simulink library "lib_Sim_CRM_16b"  (Simulink 8.8)
settings: Solver=VariableStepAuto  StartTime=0.0  StopTime=10.0  RelTol=1e-3
undefined symbols (not defined in the file): CRM
libraries: simulink x1
settings Model: Creator=cava_da  LastModifiedBy=cava_da

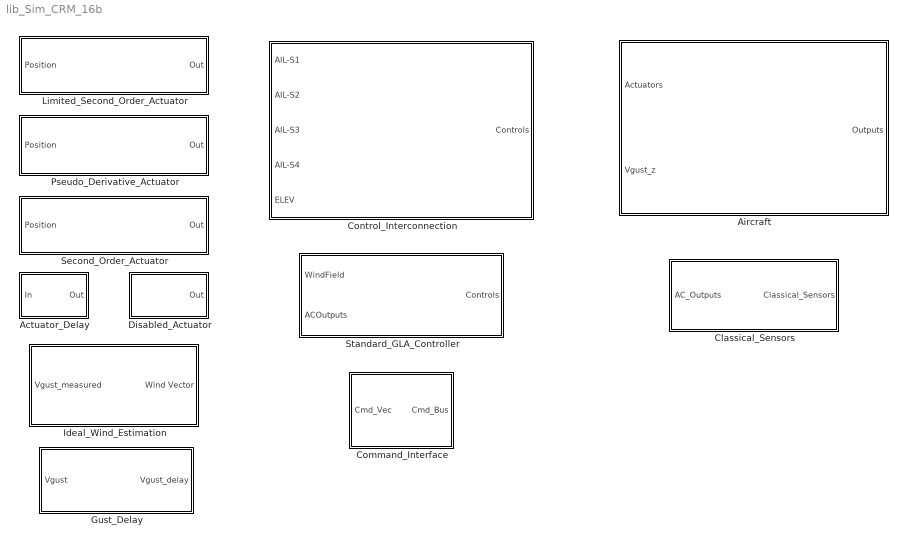
== system lib_Sim_CRM_16b ==
  Actuator_Delay : Subsystem  mask(Actuator Delay){Act_Delay=CRM.Actuators.Global_Delay}
      mask prompts: Act_Delay "Insert actuator delay [s]"
      mask help: Applies a transport delay to actuator commands.
      mask Display:
      | port_label('input', 1, '')
      | port_label('output',1, '')
  Aircraft : Subsystem  mask(Aircraft model){modelName=CRM.Aircraft}
      mask prompts: modelName "Insert name of model parameter struct (e.g. CRM.Aircraft):"
      mask help:
      | Contains the state-space model of the aircraft, separates the outputs and
      | measurements, as specified.
      mask Display:
      | port_label('input', 2, 'Gust')
      | port_label('input', 1, 'Actuators')
      | port_label('output', 1, 'Outputs')
  Classical_Sensors : Subsystem
  Command_Interface : Subsystem
  Control_Interconnection : Subsystem  mask(Control interconnection block){}
      mask help:
      | Accepts actuator states in the form of a bus containing position, rate,
      | and acceleration (delta, deltadot, delta2dot, respectively) for each
      | actuator, and rearranges them in the order required by the model.
      mask Display:
      | image(imread('plane_actuators_color.png'))
      | port_label('output', 1, 'Actuators')
      | port_label('input', 1, 'S1')
      | port_label('input', 2, 'S2')
      | port_label('input', 3, 'S3')
      | port_label('input', 4, 'S4')
      | port_label('input', 5, 'ELEV')
  Disabled_Actuator : Subsystem  mask(Disabled Actuator){}
      mask help:
      | Generates a bus containing actuator position,
      | rate, and acceleration equal to zero.
      mask Display:
      | port_label('output',1, 'Pos/Rate/Acc')
      | text(0.5,0.1, 'DA', 'horizontalAlignment', 'center')
  Gust_Delay : Subsystem  mask(Gust delay block){weName=CRM.WindEst}
      mask prompts: weName "Insert the wind estimation struct (e.g. CRM.WindEst):"
      mask help:
      | Delays the gust input so that it 'arrives' at the aircraft nose with the
      | appropriate delay w.r.t. the LIDAR/Wind Estimator prediction.
      mask Display:
      | port_label('input', 1, 'Measured gust')
      | port_label('output', 1, 'Delayed gust')
  Ideal_Wind_Estimation : Subsystem  mask(Wind Estimation Block){weName=CRM.WindEst}
      mask prompts: weName "Insert the wind estimation struct (e.g. CRM.WindEst):"
      mask help:
      | Accepts wind speed (measured by LIDAR) and generates the delayed vector of
      | estimated wind speeds.
      | The wind vector is ordered from oldest (i.e. at aircraft position) to newest
      | (i.e. currently measured by LIDAR).
      mask Display:
      | port_label('input', 1, 'Measured Wind')
      | port_label('output', 1, 'Wind Vector')
  Limited_Second_Order_Actuator : Subsystem  mask(Second-Order Actuator){actuatorName=CRM.Actuators.OuterAileron}
      mask prompts: actuatorName "Insert actuator struct (e.g. CRM.Actuators.OuterAileron):"
      mask help:
      | Accepts a commanded actuator position, and
      | generates a bus containing actuator position,
      | rate, and acceleration.
      |
      | This block uses a 2nd-order linear system to
      | approximate an actuation loop.
      mask Display:
      | port_label('input', 1, 'Commanded Pos')
      | port_label('output',1, 'Pos/Rate/Acc')
      | text(0.5,0.1, 'SO-LIM', 'horizontalAlignment', 'center')
  Pseudo_Derivative_Actuator : Subsystem  mask(Pseudo-derivative Actuator){actuatorName=CRM.Actuators.OuterAileron}
      mask prompts: actuatorName "Insert actuator struct (e.g. CRM.Actuators.Aileron):"
      mask help:
      | Accepts a commanded actuator position, and
      | generates a bus containing actuator position,
      | rate, and acceleration.
      |
      | This block uses 2 pseudo-derivatives to approximate this.
      mask Display:
      | port_label('input', 1, 'Commanded Pos')
      | port_label('output',1, 'Pos/Rate/Acc')
      | text(0.5,0.1, 'PD', 'horizontalAlignment', 'center')
  Second_Order_Actuator : Subsystem  mask(Second-Order Actuator){actuatorName=CRM.Actuators.OuterAileron}
      mask prompts: actuatorName "Insert actuator struct (e.g. CRM.Actuators.OuterAileron):"
      mask help:
      | Accepts a commanded actuator position, and
      | generates a bus containing actuator position,
      | rate, and acceleration.
      |
      | This block uses a 2nd-order linear system to
      | approximate an actuation loop.
      mask Display:
      | port_label('input', 1, 'Commanded Pos')
      | port_label('output',1, 'Pos/Rate/Acc')
      | text(0.5,0.1, 'SO', 'horizontalAlignment', 'center')
  Standard_GLA_Controller : Subsystem  mask(Simple Gust Load Alleviation Controller Block){glaName=CRM.GLA}
      mask prompts: glaName "Insert the GLA structure (e.g. CRM.GLA):"
      mask help:
      | Calculates control inputs based on measured variables, such as the lidar wind field.
      | This block assumes that the controller is contained in a single discrete state-space system.
      | The output contains 3 signals, in the following order:
      |    Inner Aileron, Outer Aileron, Elevator.
      | If the controller does not use one or more of them, it is automatically set to 0.
      mask Display:
      | port_label('input', 2, 'A/C Outputs')
      | port_label('input', 1, 'Wind Field')
      | port_label('output', 1, 'Controls')

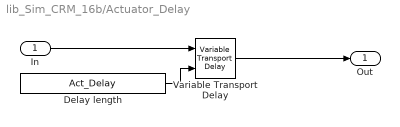
== system lib_Sim_CRM_16b/Actuator_Delay ==
  In : Inport
  Delay length : Constant  Value=Act_Delay
  Variable Transport Delay : VariableTransportDelay  MaximumDelay=Act_Delay  ZeroDelay=on
  Out : Outport
  wires:
  Variable Transport Delay/1 -> Out/1
  In/1 -> Variable Transport Delay/1
  Delay length/1 -> Variable Transport Delay/2

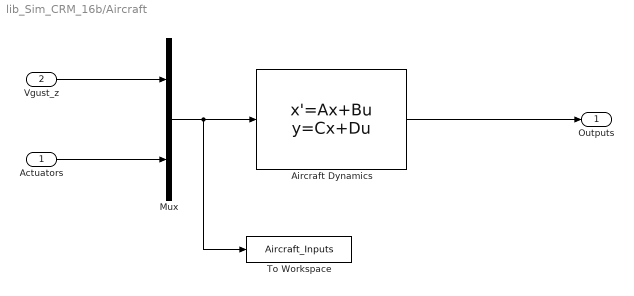
== system lib_Sim_CRM_16b/Aircraft ==
  Actuators : Inport
  Vgust_z : Inport  Port=2
  Aircraft Dynamics : StateSpace  A=modelName.linear_sys.A  B=modelName.linear_sys.B  C=[modelName.C_sensors; modelName.C_outputs]  D=[modelName.D_sensors; modelName.D_outputs]  X0=0
  Mux : Mux  Inputs=2
  To Workspace : ToWorkspace  VariableName=Aircraft_Inputs  SaveFormat=Structure With Time  SampleTime=-1
      settings: Decimation=SimConfig.Logging.DecimationFactor
  Outputs : Outport
  wires:
  Mux/1 -> To Workspace/1, Aircraft Dynamics/1
  Aircraft Dynamics/1 -> Outputs/1
  Vgust_z/1 -> Mux/1
  Actuators/1 -> Mux/2

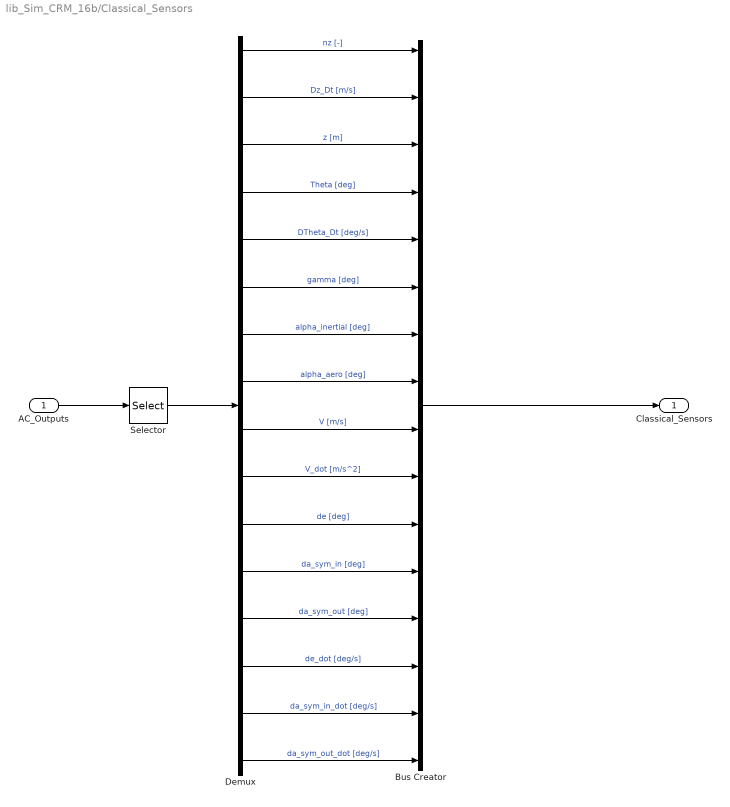
== system lib_Sim_CRM_16b/Classical_Sensors ==
  AC_Outputs : Inport
  Bus Creator : BusCreator  Inputs=16
  Demux : Demux  Outputs=16
  Selector : Selector  IndexOptions=Index vector (dialog)  Indices=1:CRM.Sensors.Classical.Num_Signals  OutputSizes=1
  Classical_Sensors : Outport
  wires:
  AC_Outputs/1 -> Selector/1
  Selector/1 -> Demux/1
  Demux/1 -> Bus Creator/1  "nz [-]"
  Demux/6 -> Bus Creator/6  "gamma [deg]"
  Demux/5 -> Bus Creator/5  "DTheta_Dt [deg/s]"
  Demux/7 -> Bus Creator/7  "alpha_inertial [deg]"
  Demux/4 -> Bus Creator/4  "Theta [deg]"
  Demux/8 -> Bus Creator/8  "alpha_aero [deg]"
  Demux/3 -> Bus Creator/3  "z [m]"
  Demux/9 -> Bus Creator/9  "V [m/s]"
  Demux/2 -> Bus Creator/2  "Dz_Dt [m/s]"
  Demux/10 -> Bus Creator/10  "V_dot [m/s^2]"
  Demux/11 -> Bus Creator/11  "de [deg]"
  Demux/12 -> Bus Creator/12  "da_sym_in [deg]"
  Demux/13 -> Bus Creator/13  "da_sym_out [deg]"
  Demux/14 -> Bus Creator/14  "de_dot [deg/s]"
  Demux/15 -> Bus Creator/15  "da_sym_in_dot [deg/s]"
  Demux/16 -> Bus Creator/16  "da_sym_out_dot [deg/s]"
  Bus Creator/1 -> Classical_Sensors/1

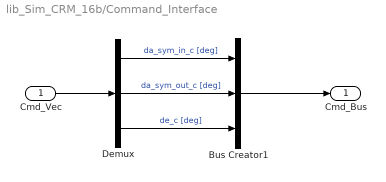
== system lib_Sim_CRM_16b/Command_Interface ==
  Cmd_Vec : Inport
  Bus Creator1 : BusCreator  Inputs=3
  Demux : Demux  Outputs=3
  Cmd_Bus : Outport
  wires:
  Demux/2 -> Bus Creator1/2  "da_sym_out_c [deg]"
  Demux/1 -> Bus Creator1/1  "da_sym_in_c [deg]"
  Demux/3 -> Bus Creator1/3  "de_c [deg]"
  Cmd_Vec/1 -> Demux/1
  Bus Creator1/1 -> Cmd_Bus/1

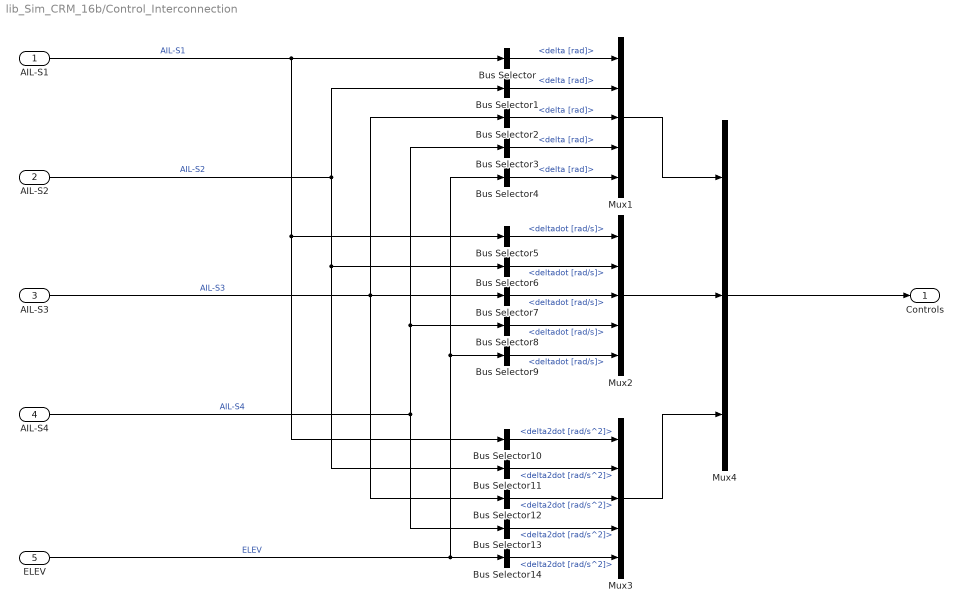
== system lib_Sim_CRM_16b/Control_Interconnection ==
  AIL-S1 : Inport
  AIL-S2 : Inport  Port=2
  AIL-S3 : Inport  Port=3
  AIL-S4 : Inport  Port=4
  ELEV : Inport  Port=5
  Bus Selector{,1..4} (5 alike) : BusSelector  OutputSignals=delta [rad]
  Bus Selector{10..14} (5 alike) : BusSelector  OutputSignals=delta2dot [rad/s^2]
  Bus Selector{5..9} (5 alike) : BusSelector  OutputSignals=deltadot [rad/s]
  Mux1 : Mux  Inputs=5
  Mux2 : Mux  Inputs=5
  Mux3 : Mux  Inputs=5
  Mux4 : Mux  Inputs=3
  Controls : Outport
  wires:
  Mux2/1 -> Mux4/2
  Mux1/1 -> Mux4/1
  Mux3/1 -> Mux4/3
  Bus Selector14/1 -> Mux3/5  "<delta2dot [rad/s^2]>"
  Bus Selector13/1 -> Mux3/4  "<delta2dot [rad/s^2]>"
  Bus Selector12/1 -> Mux3/3  "<delta2dot [rad/s^2]>"
  Bus Selector11/1 -> Mux3/2  "<delta2dot [rad/s^2]>"
  Bus Selector10/1 -> Mux3/1  "<delta2dot [rad/s^2]>"
  Bus Selector9/1 -> Mux2/5  "<deltadot [rad/s]>"
  Bus Selector8/1 -> Mux2/4  "<deltadot [rad/s]>"
  Bus Selector7/1 -> Mux2/3  "<deltadot [rad/s]>"
  Bus Selector6/1 -> Mux2/2  "<deltadot [rad/s]>"
  Bus Selector5/1 -> Mux2/1  "<deltadot [rad/s]>"
  Bus Selector4/1 -> Mux1/5  "<delta [rad]>"
  Bus Selector3/1 -> Mux1/4  "<delta [rad]>"
  Bus Selector2/1 -> Mux1/3  "<delta [rad]>"
  Bus Selector1/1 -> Mux1/2  "<delta [rad]>"
  Bus Selector/1 -> Mux1/1  "<delta [rad]>"
  AIL-S1/1 -> Bus Selector/1, Bus Selector5/1, Bus Selector10/1  "AIL-S1"
  AIL-S2/1 -> Bus Selector1/1, Bus Selector6/1, Bus Selector11/1  "AIL-S2"
  AIL-S3/1 -> Bus Selector2/1, Bus Selector7/1, Bus Selector12/1  "AIL-S3"
  Mux4/1 -> Controls/1
  AIL-S4/1 -> Bus Selector3/1, Bus Selector8/1, Bus Selector13/1  "AIL-S4"
  ELEV/1 -> Bus Selector4/1, Bus Selector9/1, Bus Selector14/1  "ELEV"

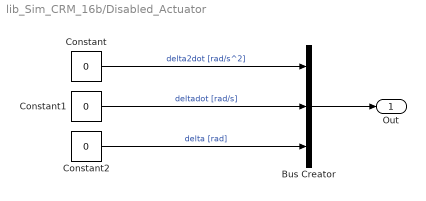
== system lib_Sim_CRM_16b/Disabled_Actuator ==
  Bus Creator : BusCreator  Inputs=3
  Constant : Constant  Value=0
  Constant1 : Constant  Value=0
  Constant2 : Constant  Value=0
  Out : Outport
  wires:
  Constant2/1 -> Bus Creator/3  "delta [rad]"
  Constant1/1 -> Bus Creator/2  "deltadot [rad/s]"
  Constant/1 -> Bus Creator/1  "delta2dot [rad/s^2]"
  Bus Creator/1 -> Out/1

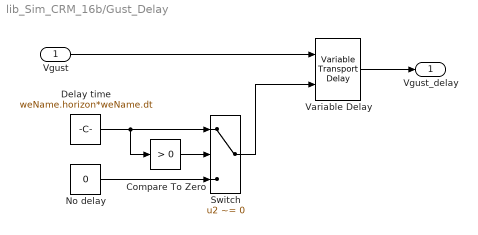
== system lib_Sim_CRM_16b/Gust_Delay ==
  Vgust : Inport
  Compare To Zero : simulink/Logic and Bit Operations/Compare To Zero  relop=>  OutDataTypeStr=uint8  ZeroCross=off
  Delay time : Constant  Value=weName.horizon*weName.dt
  No delay : Constant  Value=0
  Switch : Switch  Criteria=u2 ~= 0
  Variable Delay : VariableTransportDelay  MaximumDelay=10  MaximumPoints=1024*15  ZeroDelay=on  TransDelayFeedthrough=on
  Vgust_delay : Outport
  wires:
  Delay time/1 -> Switch/1, Compare To Zero/1
  Vgust/1 -> Variable Delay/1
  Variable Delay/1 -> Vgust_delay/1
  No delay/1 -> Switch/3
  Compare To Zero/1 -> Switch/2
  Switch/1 -> Variable Delay/2

== system lib_Sim_CRM_16b/Ideal_Wind_Estimation ==
  Vgust_measured : Inport
  Wind Estimator : DiscreteStateSpace  A=weName.A  B=weName.B  C=weName.C  D=weName.D  SampleTime=weName.dt
  Zero-Order Hold : ZeroOrderHold  SampleTime=weName.dt
  Wind Vector : Outport
  wires:
  Zero-Order Hold/1 -> Wind Estimator/1
  Wind Estimator/1 -> Wind Vector/1
  Vgust_measured/1 -> Zero-Order Hold/1

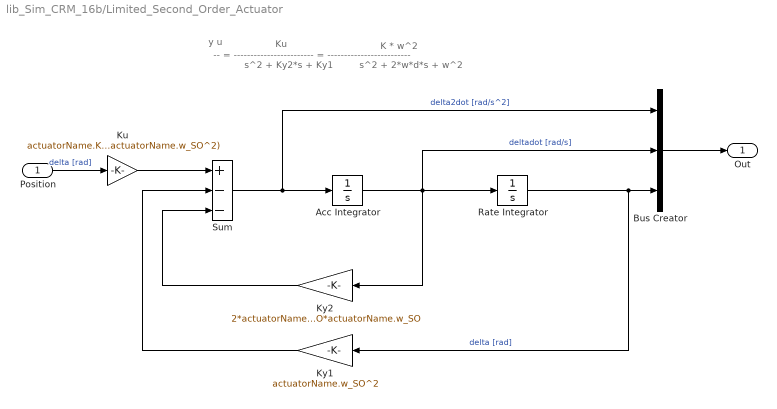
== system lib_Sim_CRM_16b/Limited_Second_Order_Actuator ==
  note: s^2 + 2*w*d*s + w^2
  note: K * w^2
  note: s^2 + Ky2*s + Ky1
  note: Ku
  note: -- = ------------------------ = -------------------------
  note: y
      |
      | u
  Position : Inport
  Acc Integrator : Integrator  LimitOutput=on  UpperSaturationLimit=actuatorName.rateLim  LowerSaturationLimit=-actuatorName.rateLim
  Bus Creator : BusCreator  Inputs=3
  Ku : Gain  Gain=actuatorName.K_st * (actuatorName.w_SO^2)
  Ky1 : Gain  Gain=actuatorName.w_SO^2
  Ky2 : Gain  Gain=2*actuatorName.d_SO*actuatorName.w_SO
  Rate Integrator : Integrator  LimitOutput=on  UpperSaturationLimit=actuatorName.posLim  LowerSaturationLimit=-actuatorName.posLim
  Sum : Sum  Inputs=+--
  Out : Outport
  wires:
  Ku/1 -> Sum/1
  Ky1/1 -> Sum/2
  Ky2/1 -> Sum/3
  Rate Integrator/1 -> Bus Creator/3, Ky1/1  "delta [rad]"
  Acc Integrator/1 -> Rate Integrator/1, Bus Creator/2, Ky2/1  "deltadot [rad/s]"
  Sum/1 -> Bus Creator/1, Acc Integrator/1  "delta2dot [rad/s^2]"
  Position/1 -> Ku/1  "delta [rad]"
  Bus Creator/1 -> Out/1

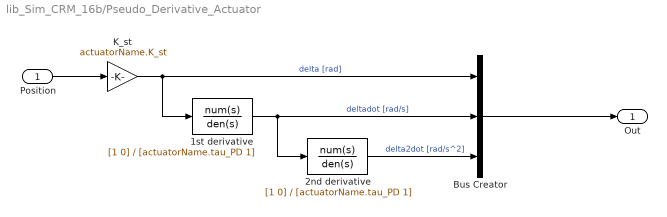
== system lib_Sim_CRM_16b/Pseudo_Derivative_Actuator ==
  Position : Inport
  1st derivative : TransferFcn  Numerator=[1 0]  Denominator=[actuatorName.tau_PD 1]
  2nd derivative : TransferFcn  Numerator=[1 0]  Denominator=[actuatorName.tau_PD 1]
  Bus Creator : BusCreator  Inputs=3
  K_st : Gain  Gain=actuatorName.K_st
  Out : Outport
  wires:
  1st derivative/1 -> 2nd derivative/1, Bus Creator/2  "deltadot [rad/s]"
  Position/1 -> K_st/1
  2nd derivative/1 -> Bus Creator/3  "delta2dot [rad/s^2]"
  Bus Creator/1 -> Out/1
  K_st/1 -> 1st derivative/1, Bus Creator/1  "delta [rad]"

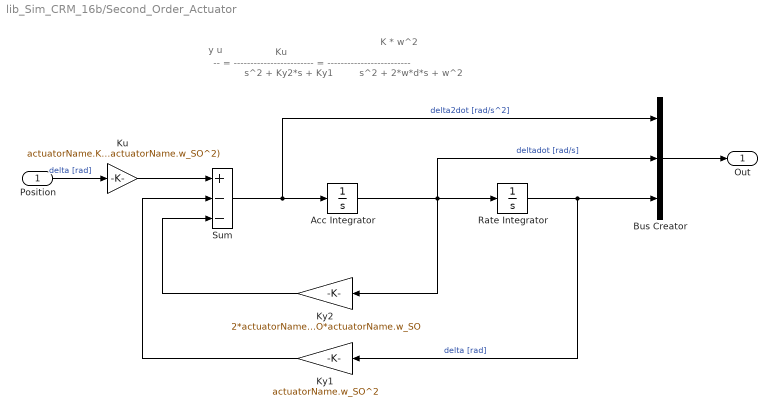
== system lib_Sim_CRM_16b/Second_Order_Actuator ==
  note: y
      |
      | u
  note: -- = ------------------------ = -------------------------
  note: Ku
  note: s^2 + Ky2*s + Ky1
  note: K * w^2
  note: s^2 + 2*w*d*s + w^2
  Position : Inport
  Acc Integrator : Integrator
  Bus Creator : BusCreator  Inputs=3
  Ku : Gain  Gain=actuatorName.K_st * (actuatorName.w_SO^2)
  Ky1 : Gain  Gain=actuatorName.w_SO^2
  Ky2 : Gain  Gain=2*actuatorName.d_SO*actuatorName.w_SO
  Rate Integrator : Integrator
  Sum : Sum  Inputs=+--
  Out : Outport
  wires:
  Bus Creator/1 -> Out/1
  Position/1 -> Ku/1  "delta [rad]"
  Sum/1 -> Acc Integrator/1, Bus Creator/1  "delta2dot [rad/s^2]"
  Acc Integrator/1 -> Rate Integrator/1, Ky2/1, Bus Creator/2  "deltadot [rad/s]"
  Rate Integrator/1 -> Ky1/1, Bus Creator/3  "delta [rad]"
  Ky2/1 -> Sum/3
  Ky1/1 -> Sum/2
  Ku/1 -> Sum/1

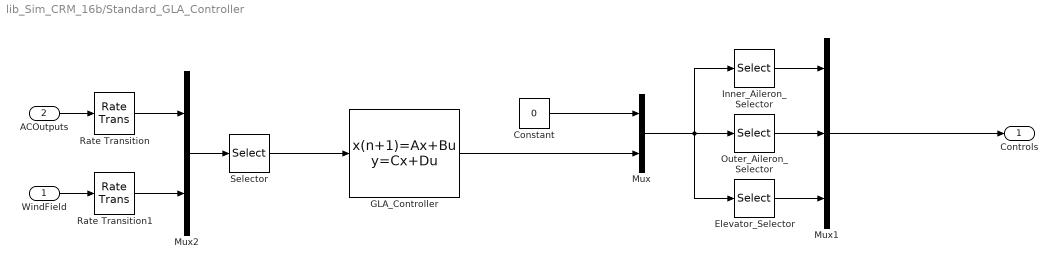
== system lib_Sim_CRM_16b/Standard_GLA_Controller ==
  WindField : Inport
  ACOutputs : Inport  Port=2
  Constant : Constant  Value=0
  Elevator_Selector : Selector  IndexMode=Zero-based  IndexOptions=Index vector (dialog)  Indices=[glaName.de_idx]  OutputSizes=1
  GLA_Controller : DiscreteStateSpace  A=glaName.A  B=glaName.B  C=glaName.C  D=glaName.D  SampleTime=glaName.dt
  Inner_Aileron_Selector : Selector  IndexMode=Zero-based  IndexOptions=Index vector (dialog)  Indices=[glaName.dain_idx]  OutputSizes=1
  Mux : Mux  Inputs=2
  Mux1 : Mux  Inputs=3
  Mux2 : Mux  Inputs=2
  Outer_Aileron_Selector : Selector  IndexMode=Zero-based  IndexOptions=Index vector (dialog)  Indices=[glaName.daout_idx]  OutputSizes=1
  Rate Transition : RateTransition  OutPortSampleTime=glaName.dt
  Rate Transition1 : RateTransition  OutPortSampleTime=glaName.dt
  Selector : Selector  IndexOptions=Index vector (dialog)  Indices=glaName.measure_idx  OutputSizes=1
  Controls : Outport
  wires:
  Mux2/1 -> Selector/1
  GLA_Controller/1 -> Mux/2
  Constant/1 -> Mux/1
  Mux/1 -> Outer_Aileron_Selector/1, Inner_Aileron_Selector/1, Elevator_Selector/1
  Outer_Aileron_Selector/1 -> Mux1/2
  Elevator_Selector/1 -> Mux1/3
  Inner_Aileron_Selector/1 -> Mux1/1
  Rate Transition/1 -> Mux2/1
  Rate Transition1/1 -> Mux2/2
  WindField/1 -> Rate Transition1/1
  ACOutputs/1 -> Rate Transition/1
  Selector/1 -> GLA_Controller/1
  Mux1/1 -> Controls/1
